simulink model "Matlab_Function"  (R2021a)
settings: Solver=FixedStepDiscrete  StartTime=0.0  StopTime=inf  FixedStep=1e-3  RelTol=1e-3  EnableMultiTasking=on
libraries: arduinolib x9, simulink x1
settings Model: SILPILModeSetting=veronly  ExtModeTrigDuration=2  Creator=Admin  LastModifiedBy=Admin
settings OptimizationCC: EnhancedBackFolding=on  PassReuseOutputArgsAs=Individual arguments  ZeroExternalMemoryAtStartup=off  ZeroInternalMemoryAtStartup=off  MaxStackSize=64  OptimizeBlockOrder=speed  DifferentSizesBufferReuse=on  OptimizationCustomize=off  EfficientTunableParamExpr=on
settings DebuggingCC: ParameterTunabilityLossMsg=error
settings HardwareCC: ProdBitPerInt=16  ProdBitPerPointer=16  ProdBitPerSizeT=16  ProdBitPerPtrDiffT=16  ProdLargestAtomicFloat=None  ProdWordSize=8  ProdHWDeviceType=Atmel->AVR
settings SFSimCC: MATLABDynamicMemAlloc=off
settings RTWCC: SystemTargetFile=ert.tlc  HardwareBoard=Arduino Uno  TemplateMakefile=ert_default_tmf  Toolchain=Arduino AVR  BuildConfiguration=Faster Runs
settings CodeAppCC: ForceParamTrailComments=on  IgnoreCustomStorageClasses=off  OperatorAnnotations=on  SimulinkDataObjDesc=on  SFDataObjDesc=on  InsertBlockDesc=on
settings ERTTargetCC: SupportContinuousTime=on  SupportVariableSizeSignals=on  ExtModeStaticAllocSize=250

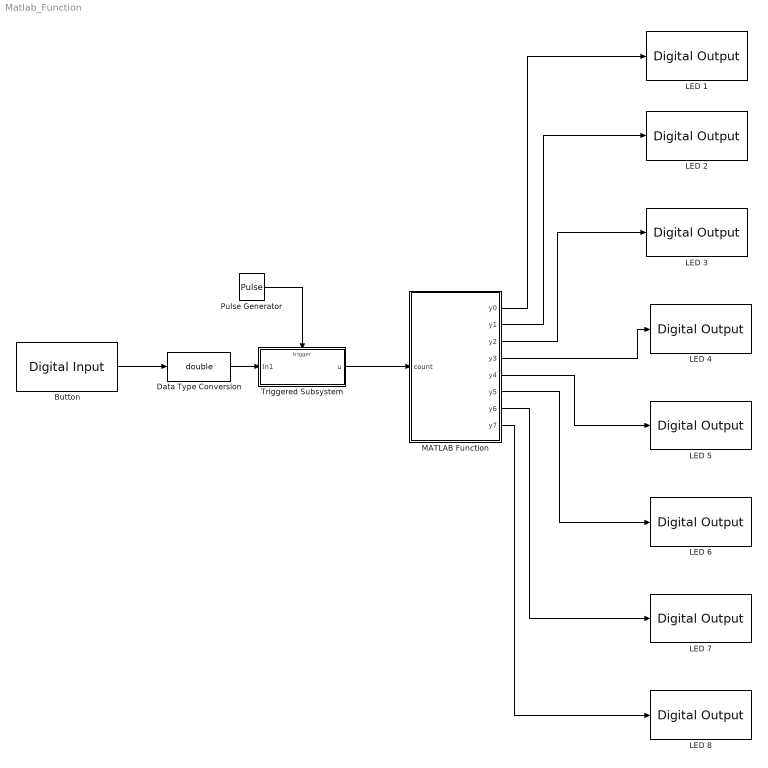
== system Matlab_Function ==
  Button : arduinolib/Digital Input  pinNumber=2  mode=Input Pullup  Direction=input  SampleTime=1e-3  blockPlatform=arduino
  Data Type Conversion : DataTypeConversion  OutDataTypeStr=double
  LED 1 : arduinolib/Digital Output  pinNumber=10  Direction=output  blockPlatform=arduino
  LED 2 : arduinolib/Digital Output  pinNumber=9  Direction=output  blockPlatform=arduino
  LED 3 : arduinolib/Digital Output  pinNumber=8  Direction=output  blockPlatform=arduino
  LED 4 : arduinolib/Digital Output  pinNumber=7  Direction=output  blockPlatform=arduino
  LED 5 : arduinolib/Digital Output  pinNumber=6  Direction=output  blockPlatform=arduino
  LED 6 : arduinolib/Digital Output  pinNumber=5  Direction=output  blockPlatform=arduino
  LED 7 : arduinolib/Digital Output  pinNumber=4  Direction=output  blockPlatform=arduino
  LED 8 : arduinolib/Digital Output  pinNumber=3  Direction=output  blockPlatform=arduino
  MATLAB Function : MATLAB Function  TreatAsAtomicUnit=on
  Pulse Generator : DiscretePulseGenerator  Period=500  PulseWidth=250  SampleTime=1e-3
  "Triggered Subsystem " : Subsystem  TreatAsAtomicUnit=on
  wires:
  Button/1 -> Data Type Conversion/1
  Pulse Generator/1 -> "Triggered Subsystem "/Trigger
  Data Type Conversion/1 -> "Triggered Subsystem "/1(In1)
  MATLAB Function/1(y0) -> LED 1/1
  MATLAB Function/2(y1) -> LED 2/1
  MATLAB Function/3(y2) -> LED 3/1
  MATLAB Function/4(y3) -> LED 4/1
  MATLAB Function/5(y4) -> LED 5/1
  MATLAB Function/6(y5) -> LED 6/1
  MATLAB Function/7(y6) -> LED 7/1
  MATLAB Function/8(y7) -> LED 8/1
  "Triggered Subsystem "/1(u) -> MATLAB Function/1(count)

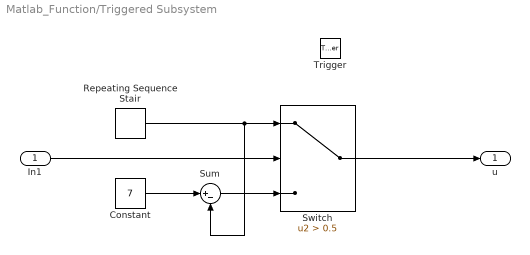
== system Matlab_Function/Triggered Subsystem  ==
  In1 : Inport
  Trigger : TriggerPort  VariantControl=(inherit)
  Constant : Constant  Value=7
  Repeating Sequence Stair : simulink/Sources/Repeating Sequence Stair  OutValues=[0 1 2 3 4 5 6 7]  tsamp=-1  OutMin=[]  OutMax=[]  OutDataTypeStr=double  OutputDataTypeScalingMode=double  OutDataType=fixdt(0,8)  ConRadixGroup=Best Precision: Vector-wise  OutScaling=2^-12
  Sum : Sum  Inputs=|+-  AccumDataTypeStr=double
  Switch : Switch  Criteria=u2 > Threshold  Threshold=0.5
  u : Outport
  wires:
  In1/1 -> Switch/2
  Repeating Sequence Stair/1 -> Sum/2, Switch/1
  Switch/1 -> u/1
  Constant/1 -> Sum/1
  Sum/1 -> Switch/3

== matlab function Matlab_Function/MATLAB Function ==
  data: count input; y0 output; y1 output; y2 output; y3 output; y4 output; y5 output; y6 output; y7 output
function [y0,y1,y2,y3,y4,y5,y6,y7] = LED_out(count)

y0 =false;y1 =false;y2 =false;y3 =false;y4 =false;y5 =false;y6 =false;y7 =false;
if count == 0
    y0 = true;
else 
    if count == 1
        y1 = true;
    else
        if count == 2
            y2 = true;
        else
            if count == 3
                y3 = true;
            else
                if count == 4
                    y4 = true;
                else
                    if count == 5
                        y5 = true;
                    else
                        if count == 6
                            y6 = true;
                        else
                            if count == 7
                                y7 = true;
                            end
                        end
                    end
                end
            end
        end
    end
end
